simulink subsystem "TractionControl_subsysref"  (R2020a)
settings: Solver=VariableStepAuto  StartTime=0.0  StopTime=10.0  RelTol=1e-3
settings Model: Creator=Kiera  LastModifiedBy=Kiera

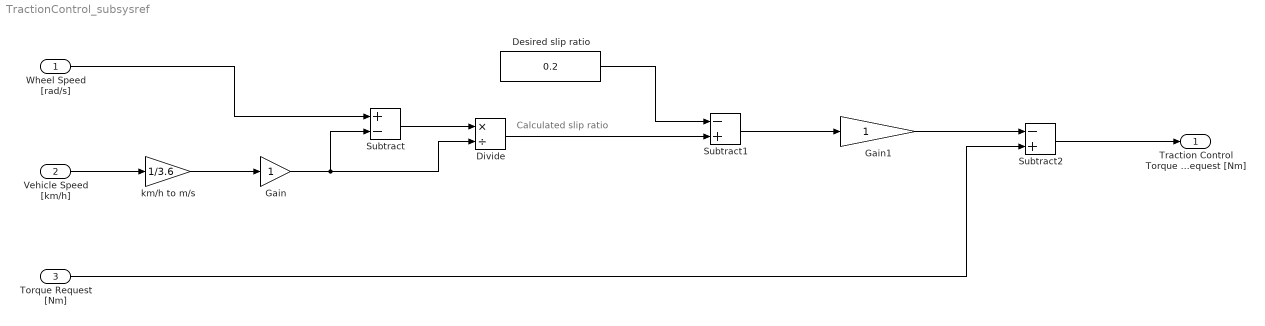
== system TractionControl_subsysref ==
  note: Calculated slip ratio
  Wheel Speed [rad/s] : Inport
  Vehicle Speed [km/h] : Inport  Port=2
  Torque Request [Nm] : Inport  Port=3
  Desired slip ratio : Constant  Value=0.2
  Divide : Product  Inputs=*/
  Gain : Gain
  Gain1 : Gain
  Subtract : Sum  Inputs=+-
  Subtract1 : Sum  Inputs=-+
  Subtract2 : Sum  Inputs=-+
  km/h to m/s : Gain  Gain=1/3.6
  Traction Control Torque Request [Nm] : Outport  VectorParamsAs1DForOutWhenUnconnected=off
  wires:
  Gain/1 -> Divide/2, Subtract/2
  km/h to m/s/1 -> Gain/1
  Subtract/1 -> Divide/1
  Vehicle Speed [km/h]/1 -> km/h to m/s/1
  Wheel Speed [rad/s]/1 -> Subtract/1
  Torque Request [Nm]/1 -> Subtract2/2
  Desired slip ratio/1 -> Subtract1/1
  Gain1/1 -> Subtract2/1
  Subtract1/1 -> Gain1/1
  Divide/1 -> Subtract1/2
  Subtract2/1 -> Traction Control Torque Request [Nm]/1
